simulink model "main_WU_motion"  (R2023a)
settings: Solver=VariableStepAuto  StartTime=0.0  StopTime=3.88  RelTol=1e-9  AbsTol=1e-9  EnableMultiTasking=on
values from neighbouring files (symbols this model uses):
  a_el = [r_ej,h_ej,r_ej]    [data.m]    (also in fo_python_to_matlab.m = [ax,ay,az])
  akt_GH = rand(1,13)*1    [inverse_dynamics.m]    (also in odvozeni_svaly.m = sym('akt_GH',[1 N_GH]))
  akt_ST = rand(1,13)*1    [inverse_dynamics.m]    (also in odvozeni_svaly.m = sym('akt_ST',[1 N_ST]))
  ccom = [-0.0110972, 0.00637508, 0.0541825]    [data.m]    (also in fo_python_to_matlab.m = [ccomx, ccomy, ccomz]; mm_python_to_matlab.m = [ccomx, ccomy, ccomz])
  cI = [5.75482e-05, 6.05521e-05, 1.05345e-05,-1.27405e-05, 1.65861e-05, 4.50136e-06]    [data.m]    (also in mm_python_to_matlab.m = [cixx, ciyy, cizz, cixy, ciyz, cizx])
  cont1 = [-0.083529 -0.01368 -0.098954]-scom    [data.m]    (also in fo_python_to_matlab.m = [x_cont1,y_cont1,z_cont1])
  cont2 = [-0.105456 -0.125076 -0.075251]-scom    [data.m]    (also in fo_python_to_matlab.m = [x_cont2,y_cont2,z_cont2])
  cont_params = [k_contact, eps]    [data.m]    (also in fo_python_to_matlab.m)
  Glenohumeral_F0M = str2double(table2array(GH(:,2)))'    [data.m]
  Glenohumeral_l0 = str2double(table2array(GH(:,3)))'    [data.m]
  h_ej = 0.15    [data.m]
  hcom = [0.000389382, -0.116338, -0.00231072]    [data.m]    (also in fo_python_to_matlab.m = [hcomx, hcomy, hcomz]; mm_python_to_matlab.m = [hcomx, hcomy, hcomz])
  hI = [0.00326632, 4.34807e-05, 0.00325004,-0.000136456, -1.30958e-06, -1.14964e-05]    [data.m]    (also in mm_python_to_matlab.m = [hixx, hiyy, hizz, hixy, hiyz, hizx])
  initialConditions = zeros(1,18)    [inverse_dynamics.m]
  k_contact = 0    [data.m]
  m = [0.0370005,0.12759,0.26363]    [data.m]    (also in fo_python_to_matlab.m = [c_m,s_m,h_m]; mm_python_to_matlab.m = [c_m,s_m,h_m])
  m_el = [x_ej,y_ej,z_ej]    [data.m]    (also in fo_python_to_matlab.m = [mx, my, mz])
  p = [c,k,g]    [data.m]    (also in fo_python_to_matlab.m)
  r_ej = 0.088    [data.m]
  Scapulothoracic_F0M = str2double(table2array(ST(:,2)))'    [data.m]
  Scapulothoracic_l0 = str2double(table2array(ST(:,3)))'    [data.m]
  scom = [-0.0512948, -0.0367122, -0.0430756]    [data.m]    (also in fo_python_to_matlab.m = [scomx, scomy, scomz]; mm_python_to_matlab.m = [scomx, scomy, scomz])
  sI = [0.00020065, 0.000202939, 0.000227237,-4.55661e-05, -7.53511e-05, -7.42694e-05]    [data.m]    (also in mm_python_to_matlab.m = [sixx, siyy, sizz, sixy, siyz, sizx])
  T_c = [-0.01433 0.02007 0.135535]    [data.m]    (also in fo_python_to_matlab.m = [T_cx,T_cy,T_cz]; mm_python_to_matlab.m = [T_cx,T_cy,T_cz]; odvozeni_svaly.m)
  T_d = 1e-20    [data.m]
  T_s = [-0.00955 -0.034 0.009]    [data.m]    (also in fo_python_to_matlab.m = [T_sx,T_sy,T_sz]; mm_python_to_matlab.m = [T_sx,T_sy,T_sz]; odvozeni_svaly.m)
  T_t = [0.006325 0.00693 0.025465]    [data.m]    (also in fo_python_to_matlab.m = [T_tx, T_ty, T_tz]; odvozeni_svaly.m)
  x_ej = -0.03    [data.m]
  y_ej = -0.1    [data.m]
  z_ej = 0.05    [data.m]
undefined symbols (not defined in the file or in its folder): phi_0, r_0, r_10, r_20, X, Y, Z
libraries: sm_lib x165, nesl_utility x96
(part 1 of 5)
settings Model: Creator=zoufi  LastModifiedBy=zoufaond
settings SolverCC: AutoScaleAbsTol=off  AlgebraicLoopSolver=TrustRegion  MaxZcPerStep=1
settings DataIOCC: LimitDataPoints=on  MaxDataPoints=10000
settings OptimizationCC: ReuseModelBlockBuffer=off  LifeSpan=inf
settings DebuggingCC: UnconnectedInputMsg=warning  UnconnectedOutputMsg=warning  UnconnectedLineMsg=warning  AllowSymbolicDim=off  SubsystemReferenceDiagnosticForUnitTest=warning  SFUnexpectedBacktrackingDiag=warning  SFNoUnconditionalDefaultTransitionDiag=warning  SFExecutionAtInitializationDiag=none  ArithmeticOperatorsInVariantConditions=warning
settings ModelReferenceCC: EnableRefExpFcnMdlSchedulingChecks=on
settings SFSimCC: SimUseLocalCustomCode=off  CustomCodeUndefinedFunction=UseInterfaceOnly
settings RTWCC: RTWUseLocalCustomCode=off  DLArmComputeVersion=19.05
settings CodeAppCC: StateflowObjectComments=on
settings GRTTargetCC: TargetLangStandard=C89/C90 (ANSI)
settings ConfigComp: CovMetricSettings=dw  CovSaveCumulativeToWorkspaceVar=on  CovSaveSingleToWorkspaceVar=on  CovExternalEMLEnable=off  CovSFcnEnable=off
settings SimscapeCC: SimscapeLogType=all  SimscapeLogSimulationStatistics=on  SimscapeLogDataHistory=10000

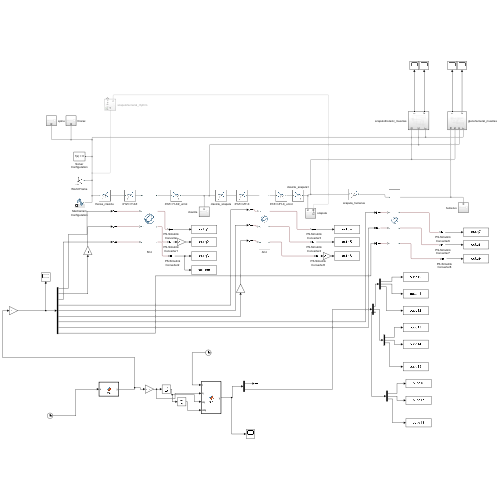
[thumbnail: Simulink's stored preview of the top-level diagram]
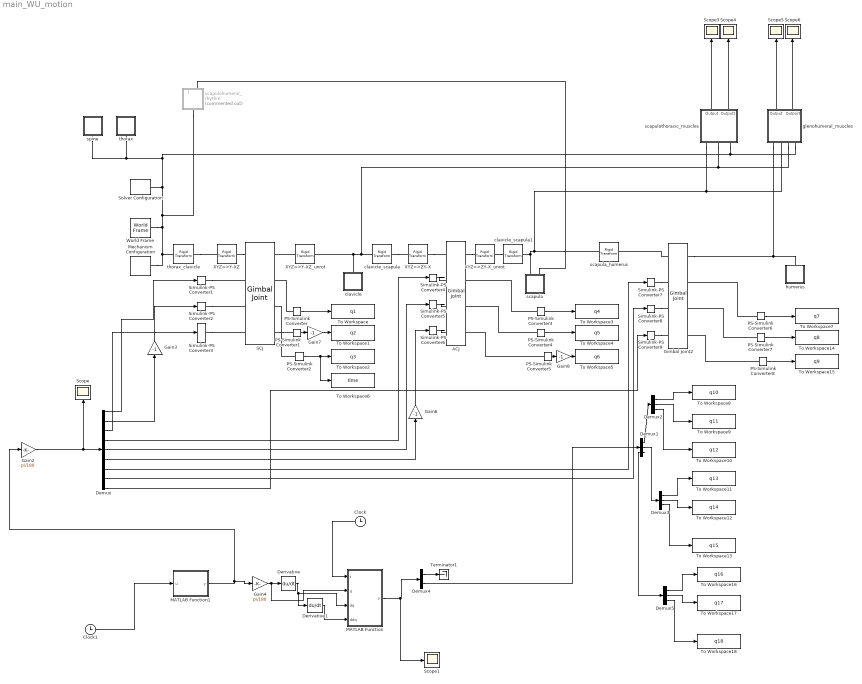
== system main_WU_motion ==
  ACJ : sm_lib/Joints/Gimbal Joint  JointMode=Normal  SenseConstraintForce=off  SenseConstraintForceX=off  SenseConstraintForceY=off  SenseConstraintForceZ=off  SenseConstraintTorque=off  SenseConstraintTorqueX=off  SenseConstraintTorqueY=off  SenseConstraintTorqueZ=off  SenseTotalForce=off  SenseTotalForceX=off  SenseTotalForceY=off  SenseTotalForceZ=off  SenseTotalTorque=off  SenseTotalTorqueX=off  SenseTotalTorqueY=off  SenseTotalTorqueZ=off  CompositeWrenchDir=FollowerOnBase  CompositeWrenchFrame=BaseFrame  RxEquilibriumPosition=0  RxEquilibriumPositionUnits=deg  RxSpringStiffness=k  RxSpringStiffnessUnits=N*m/rad  RxDampingCoefficient=c  RxDampingCoefficientUnits=N*m/(rad/s)  RxTorqueActuationMode=ComputedTorque  RxMotionActuationMode=InputMotion  RxSensePosition=off  RxSenseVelocity=off  RxSenseAcceleration=off  RxSenseTorqueForce=on  RxSenseLowerLimitTorqueForce=off  RxSenseUpperLimitTorqueForce=off  RxLowerLimitSpecify=off  RxLowerLimitBound=-90  RxLowerLimitBoundUnits=deg  RxLowerLimitStiffness=1e4  RxLowerLimitStiffnessUnits=N*m/deg  RxLowerLimitDamping=10  RxLowerLimitDampingUnits=N*m/(deg/s)  RxLowerLimitTransitionRegionWidth=0.1  RxLowerLimitTransitionRegionWidthUnits=deg  RxUpperLimitSpecify=off  RxUpperLimitBound=90  RxUpperLimitBoundUnits=deg  RxUpperLimitStiffness=1e4  RxUpperLimitStiffnessUnits=N*m/deg  RxUpperLimitDamping=10  RxUpperLimitDampingUnits=N*m/(deg/s)  RxUpperLimitTransitionRegionWidth=0.1  RxUpperLimitTransitionRegionWidthUnits=deg  RxPositionTargetSpecify=on  RxPositionTargetPriority=High  RxPositionTargetValue=initialConditions(4)  RxPositionTargetValueUnits=rad  RxVelocityTargetSpecify=off  RxVelocityTargetPriority=High  RxVelocityTargetValue=0  RxVelocityTargetValueUnits=deg/s  RyEquilibriumPosition=0  RyEquilibriumPositionUnits=deg  RySpringStiffness=k  RySpringStiffnessUnits=N*m/rad  RyDampingCoefficient=c  RyDampingCoefficientUnits=N*m/(rad/s)  RyTorqueActuationMode=ComputedTorque  RyMotionActuationMode=InputMotion  RySensePosition=off  RySenseVelocity=off  RySenseAcceleration=off  RySenseTorqueForce=on  RySenseLowerLimitTorqueForce=off  RySenseUpperLimitTorqueForce=off  RyLowerLimitSpecify=off  RyLowerLimitBound=-90  RyLowerLimitBoundUnits=deg  RyLowerLimitStiffness=1e4  RyLowerLimitStiffnessUnits=N*m/deg  RyLowerLimitDamping=10  RyLowerLimitDampingUnits=N*m/(deg/s)  RyLowerLimitTransitionRegionWidth=0.1  RyLowerLimitTransitionRegionWidthUnits=deg  RyUpperLimitSpecify=off  RyUpperLimitBound=90  RyUpperLimitBoundUnits=deg  RyUpperLimitStiffness=1e4  RyUpperLimitStiffnessUnits=N*m/deg  RyUpperLimitDamping=10  RyUpperLimitDampingUnits=N*m/(deg/s)  RyUpperLimitTransitionRegionWidth=0.1  RyUpperLimitTransitionRegionWidthUnits=deg  RyPositionTargetSpecify=on  RyPositionTargetPriority=High  RyPositionTargetValue=initialConditions(5)  RyPositionTargetValueUnits=rad  RyVelocityTargetSpecify=off  RyVelocityTargetPriority=High  RyVelocityTargetValue=0  RyVelocityTargetValueUnits=deg/s  RzEquilibriumPosition=0  RzEquilibriumPositionUnits=deg  RzSpringStiffness=k  RzSpringStiffnessUnits=N*m/rad  RzDampingCoefficient=c  RzDampingCoefficientUnits=N*m/(rad/s)  RzTorqueActuationMode=ComputedTorque  RzMotionActuationMode=InputMotion  RzSensePosition=off  RzSenseVelocity=off  RzSenseAcceleration=off  RzSenseTorqueForce=on  RzSenseLowerLimitTorqueForce=off  RzSenseUpperLimitTorqueForce=off  RzLowerLimitSpecify=off  RzLowerLimitBound=-90  RzLowerLimitBoundUnits=deg  RzLowerLimitStiffness=1e4  RzLowerLimitStiffnessUnits=N*m/deg  RzLowerLimitDamping=10  RzLowerLimitDampingUnits=N*m/(deg/s)  RzLowerLimitTransitionRegionWidth=0.1  RzLowerLimitTransitionRegionWidthUnits=deg  RzUpperLimitSpecify=off  RzUpperLimitBound=90  RzUpperLimitBoundUnits=deg  RzUpperLimitStiffness=1e4  RzUpperLimitStiffnessUnits=N*m/deg  RzUpperLimitDamping=10  RzUpperLimitDampingUnits=N*m/(deg/s)  RzUpperLimitTransitionRegionWidth=0.1  RzUpperLimitTransitionRegionWidthUnits=deg  RzPositionTargetSpecify=on  RzPositionTargetPriority=High  RzPositionTargetValue=initialConditions(6)  RzPositionTargetValueUnits=rad  RzVelocityTargetSpecify=off  RzVelocityTargetPriority=High  RzVelocityTargetValue=0  RzVelocityTargetValueUnits=deg/s
  Clock : Clock
  Clock1 : Clock
  Demux : Demux  Outputs=9
  Demux{1..3,5} (4 alike) : Demux  Outputs=3
  Demux4 : Demux  Outputs=2
  Derivative : Derivative
  Derivative1 : Derivative
  Gain2 : Gain  Gain=pi/180
  Gain{3,6..8} (4 alike) : Gain  Gain=-1
  Gain4 : Gain  Gain=pi/180
  Gimbal Joint2 : sm_lib/Joints/Gimbal Joint  JointMode=Normal  SenseConstraintForce=off  SenseConstraintForceX=off  SenseConstraintForceY=off  SenseConstraintForceZ=off  SenseConstraintTorque=off  SenseConstraintTorqueX=off  SenseConstraintTorqueY=off  SenseConstraintTorqueZ=off  SenseTotalForce=off  SenseTotalForceX=off  SenseTotalForceY=off  SenseTotalForceZ=off  SenseTotalTorque=off  SenseTotalTorqueX=off  SenseTotalTorqueY=off  SenseTotalTorqueZ=off  CompositeWrenchDir=FollowerOnBase  CompositeWrenchFrame=BaseFrame  RxEquilibriumPosition=0  RxEquilibriumPositionUnits=deg  RxSpringStiffness=k  RxSpringStiffnessUnits=N*m/rad  RxDampingCoefficient=c  RxDampingCoefficientUnits=N*m/(rad/s)  RxTorqueActuationMode=ComputedTorque  RxMotionActuationMode=InputMotion  RxSensePosition=off  RxSenseVelocity=off  RxSenseAcceleration=off  RxSenseTorqueForce=on  RxSenseLowerLimitTorqueForce=off  RxSenseUpperLimitTorqueForce=off  RxLowerLimitSpecify=off  RxLowerLimitBound=-90  RxLowerLimitBoundUnits=deg  RxLowerLimitStiffness=1e4  RxLowerLimitStiffnessUnits=N*m/deg  RxLowerLimitDamping=10  RxLowerLimitDampingUnits=N*m/(deg/s)  RxLowerLimitTransitionRegionWidth=0.1  RxLowerLimitTransitionRegionWidthUnits=deg  RxUpperLimitSpecify=off  RxUpperLimitBound=90  RxUpperLimitBoundUnits=deg  RxUpperLimitStiffness=1e4  RxUpperLimitStiffnessUnits=N*m/deg  RxUpperLimitDamping=10  RxUpperLimitDampingUnits=N*m/(deg/s)  RxUpperLimitTransitionRegionWidth=0.1  RxUpperLimitTransitionRegionWidthUnits=deg  RxPositionTargetSpecify=on  RxPositionTargetPriority=High  RxPositionTargetValue=initialConditions(4)  RxPositionTargetValueUnits=rad  RxVelocityTargetSpecify=off  RxVelocityTargetPriority=High  RxVelocityTargetValue=0  RxVelocityTargetValueUnits=deg/s  RyEquilibriumPosition=0  RyEquilibriumPositionUnits=deg  RySpringStiffness=k  RySpringStiffnessUnits=N*m/rad  RyDampingCoefficient=c  RyDampingCoefficientUnits=N*m/(rad/s)  RyTorqueActuationMode=ComputedTorque  RyMotionActuationMode=InputMotion  RySensePosition=off  RySenseVelocity=off  RySenseAcceleration=off  RySenseTorqueForce=on  RySenseLowerLimitTorqueForce=off  RySenseUpperLimitTorqueForce=off  RyLowerLimitSpecify=off  RyLowerLimitBound=-90  RyLowerLimitBoundUnits=deg  RyLowerLimitStiffness=1e4  RyLowerLimitStiffnessUnits=N*m/deg  RyLowerLimitDamping=10  RyLowerLimitDampingUnits=N*m/(deg/s)  RyLowerLimitTransitionRegionWidth=0.1  RyLowerLimitTransitionRegionWidthUnits=deg  RyUpperLimitSpecify=off  RyUpperLimitBound=90  RyUpperLimitBoundUnits=deg  RyUpperLimitStiffness=1e4  RyUpperLimitStiffnessUnits=N*m/deg  RyUpperLimitDamping=10  RyUpperLimitDampingUnits=N*m/(deg/s)  RyUpperLimitTransitionRegionWidth=0.1  RyUpperLimitTransitionRegionWidthUnits=deg  RyPositionTargetSpecify=on  RyPositionTargetPriority=High  RyPositionTargetValue=initialConditions(5)  RyPositionTargetValueUnits=rad  RyVelocityTargetSpecify=off  RyVelocityTargetPriority=High  RyVelocityTargetValue=0  RyVelocityTargetValueUnits=deg/s  RzEquilibriumPosition=0  RzEquilibriumPositionUnits=deg  RzSpringStiffness=k  RzSpringStiffnessUnits=N*m/rad  RzDampingCoefficient=c  RzDampingCoefficientUnits=N*m/(rad/s)  RzTorqueActuationMode=ComputedTorque  RzMotionActuationMode=InputMotion  RzSensePosition=off  RzSenseVelocity=off  RzSenseAcceleration=off  RzSenseTorqueForce=on  RzSenseLowerLimitTorqueForce=off  RzSenseUpperLimitTorqueForce=off  RzLowerLimitSpecify=off  RzLowerLimitBound=-90  RzLowerLimitBoundUnits=deg  RzLowerLimitStiffness=1e4  RzLowerLimitStiffnessUnits=N*m/deg  RzLowerLimitDamping=10  RzLowerLimitDampingUnits=N*m/(deg/s)  RzLowerLimitTransitionRegionWidth=0.1  RzLowerLimitTransitionRegionWidthUnits=deg  RzUpperLimitSpecify=off  RzUpperLimitBound=90  RzUpperLimitBoundUnits=deg  RzUpperLimitStiffness=1e4  RzUpperLimitStiffnessUnits=N*m/deg  RzUpperLimitDamping=10  RzUpperLimitDampingUnits=N*m/(deg/s)  RzUpperLimitTransitionRegionWidth=0.1  RzUpperLimitTransitionRegionWidthUnits=deg  RzPositionTargetSpecify=on  RzPositionTargetPriority=High  RzPositionTargetValue=initialConditions(6)  RzPositionTargetValueUnits=rad  RzVelocityTargetSpecify=off  RzVelocityTargetPriority=High  RzVelocityTargetValue=0  RzVelocityTargetValueUnits=deg/s
  MATLAB Function : MATLAB Function  TreatAsAtomicUnit=on
  MATLAB Function1 : MATLAB Function  TreatAsAtomicUnit=on
  Mechanism Configuration : sm_lib/Utilities/Mechanism Configuration  UniformGravity=Constant  GravityVector=[0 -9.80665 0]  GravityVectorUnits=m/s^2  LinearizationDelta=0.001  JointModeTransitionNonlinearIterations=2
  PS-Simulink Converter{,1..8} (9 alike) : nesl_utility/PS-Simulink Converter  PhysicalDomain=network_engine_domain  SubClassName=ps_output  LeftPortType=input  RightPortType=output  PseudoPeriodic=off  Frequencies=[]  VectorFormat=inherit  Unit=inherit  AffineConversion=off
  SCJ : sm_lib/Joints/Gimbal Joint  JointMode=Normal  SenseConstraintForce=off  SenseConstraintForceX=off  SenseConstraintForceY=off  SenseConstraintForceZ=off  SenseConstraintTorque=off  SenseConstraintTorqueX=off  SenseConstraintTorqueY=off  SenseConstraintTorqueZ=off  SenseTotalForce=off  SenseTotalForceX=off  SenseTotalForceY=off  SenseTotalForceZ=off  SenseTotalTorque=off  SenseTotalTorqueX=off  SenseTotalTorqueY=off  SenseTotalTorqueZ=off  CompositeWrenchDir=FollowerOnBase  CompositeWrenchFrame=BaseFrame  RxEquilibriumPosition=0  RxEquilibriumPositionUnits=deg  RxSpringStiffness=k  RxSpringStiffnessUnits=N*m/rad  RxDampingCoefficient=c  RxDampingCoefficientUnits=N*m/(rad/s)  RxTorqueActuationMode=ComputedTorque  RxMotionActuationMode=InputMotion  RxSensePosition=off  RxSenseVelocity=off  RxSenseAcceleration=off  RxSenseTorqueForce=on  RxSenseLowerLimitTorqueForce=off  RxSenseUpperLimitTorqueForce=off  RxLowerLimitSpecify=off  RxLowerLimitBound=-90  RxLowerLimitBoundUnits=deg  RxLowerLimitStiffness=1e4  RxLowerLimitStiffnessUnits=N*m/deg  RxLowerLimitDamping=10  RxLowerLimitDampingUnits=N*m/(deg/s)  RxLowerLimitTransitionRegionWidth=0.1  RxLowerLimitTransitionRegionWidthUnits=deg  RxUpperLimitSpecify=off  RxUpperLimitBound=90  RxUpperLimitBoundUnits=deg  RxUpperLimitStiffness=1e4  RxUpperLimitStiffnessUnits=N*m/deg  RxUpperLimitDamping=10  RxUpperLimitDampingUnits=N*m/(deg/s)  RxUpperLimitTransitionRegionWidth=0.1  RxUpperLimitTransitionRegionWidthUnits=deg  RxPositionTargetSpecify=on  RxPositionTargetPriority=High  RxPositionTargetValue=initialConditions(1)  RxPositionTargetValueUnits=rad  RxVelocityTargetSpecify=off  RxVelocityTargetPriority=High  RxVelocityTargetValue=0  RxVelocityTargetValueUnits=deg/s  RyEquilibriumPosition=0  RyEquilibriumPositionUnits=deg  RySpringStiffness=k  RySpringStiffnessUnits=N*m/rad  RyDampingCoefficient=c  RyDampingCoefficientUnits=N*m/(rad/s)  RyTorqueActuationMode=ComputedTorque  RyMotionActuationMode=InputMotion  RySensePosition=off  RySenseVelocity=off  RySenseAcceleration=off  RySenseTorqueForce=on  RySenseLowerLimitTorqueForce=off  RySenseUpperLimitTorqueForce=off  RyLowerLimitSpecify=off  RyLowerLimitBound=-90  RyLowerLimitBoundUnits=deg  RyLowerLimitStiffness=1e4  RyLowerLimitStiffnessUnits=N*m/deg  RyLowerLimitDamping=10  RyLowerLimitDampingUnits=N*m/(deg/s)  RyLowerLimitTransitionRegionWidth=0.1  RyLowerLimitTransitionRegionWidthUnits=deg  RyUpperLimitSpecify=off  RyUpperLimitBound=90  RyUpperLimitBoundUnits=deg  RyUpperLimitStiffness=1e4  RyUpperLimitStiffnessUnits=N*m/deg  RyUpperLimitDamping=10  RyUpperLimitDampingUnits=N*m/(deg/s)  RyUpperLimitTransitionRegionWidth=0.1  RyUpperLimitTransitionRegionWidthUnits=deg  RyPositionTargetSpecify=on  RyPositionTargetPriority=High  RyPositionTargetValue=initialConditions(2)  RyPositionTargetValueUnits=rad  RyVelocityTargetSpecify=off  RyVelocityTargetPriority=High  RyVelocityTargetValue=0  RyVelocityTargetValueUnits=deg/s  RzEquilibriumPosition=0  RzEquilibriumPositionUnits=deg  RzSpringStiffness=k  RzSpringStiffnessUnits=N*m/rad  RzDampingCoefficient=c  RzDampingCoefficientUnits=N*m/(rad/s)  RzTorqueActuationMode=ComputedTorque  RzMotionActuationMode=InputMotion  RzSensePosition=off  RzSenseVelocity=off  RzSenseAcceleration=off  RzSenseTorqueForce=on  RzSenseLowerLimitTorqueForce=off  RzSenseUpperLimitTorqueForce=off  RzLowerLimitSpecify=off  RzLowerLimitBound=-90  RzLowerLimitBoundUnits=deg  RzLowerLimitStiffness=1e4  RzLowerLimitStiffnessUnits=N*m/deg  RzLowerLimitDamping=10  RzLowerLimitDampingUnits=N*m/(deg/s)  RzLowerLimitTransitionRegionWidth=0.1  RzLowerLimitTransitionRegionWidthUnits=deg  RzUpperLimitSpecify=off  RzUpperLimitBound=90  RzUpperLimitBoundUnits=deg  RzUpperLimitStiffness=1e4  RzUpperLimitStiffnessUnits=N*m/deg  RzUpperLimitDamping=10  RzUpperLimitDampingUnits=N*m/(deg/s)  RzUpperLimitTransitionRegionWidth=0.1  RzUpperLimitTransitionRegionWidthUnits=deg  RzPositionTargetSpecify=on  RzPositionTargetPriority=High  RzPositionTargetValue=initialConditions(3)  RzPositionTargetValueUnits=rad  RzVelocityTargetSpecify=off  RzVelocityTargetPriority=High  RzVelocityTargetValue=0  RzVelocityTargetValueUnits=deg/s
  Scope{,1,3..6} (6 alike) : Scope
  Simulink-PS Converter{1..2,4..9} (8 alike) : nesl_utility/Simulink-PS Converter  PhysicalDomain=network_engine_domain  SubClassName=ps_input  LeftPortType=input  RightPortType=output  PseudoPeriodic=off  Frequencies=[]  NoiseDistribution=none  NoiseParameters=[]  Unit=1  AffineConversion=off  FilteringAndDerivatives=filter  SimscapeFilterOrder=2  InputFilterTimeConstant=0.001  UdotUserProvided=0
  Simulink-PS Converter3 : nesl_utility/Simulink-PS Converter  PhysicalDomain=network_engine_domain  SubClassName=ps_input  LeftPortType=input  RightPortType=output  PseudoPeriodic=off  Frequencies=[]  NoiseDistribution=none  NoiseParameters=[]  Unit=1  AffineConversion=off  FilteringAndDerivatives=filter  SimscapeFilterOrder=2  InputFilterTimeConstant=0.001  UdotUserProvided=2
  Solver Configuration : nesl_utility/Solver Configuration  PhysicalDomain=network_engine_domain  SubClassName=solver  LeftPortType=input  RightPortType=generic  Tones=[]  Harmonics=[]  SimulateNoise=off  Profile=off  UseLocalSampling=off  EnableSwitchedLinearOptims=on  FrequencyDomain=off  UseCCode=off  RelTol=0.001  AbsTol=1e-06  MinStep=1e-09  ToWorkspace=off  RevertToSquareIcSolve=off  NumHomotopyIterations=100  PhasorMode=off  PhasorModeNumHarmonics=1  ConsistencySolver=NEWTON_XTOL_AFTER_FTOL  IndexReductionMethod=DerivativeReplacement  DoDC=off  ResidualTolerance=1e-09  ConsistencyTolSource=GLOBAL  ConsistencyAbsTol=0.001  ConsistencyRelTol=0.001  ConsistencyTolFactor=0.001  UseLocalSolver=off  LocalSolverChoice=NE_BACKWARD_EULER_ADVANCER  ResolveIndetEquations=on  FunctionEvalNumThread=1  LocalSolverSampleTime=0.001  DoFixedCost=off  MaxNonlinIter=3  MaxModeIter=2  ComputeImpulses=off  ImpulseIterations=2  LinearAlgebra=Sparse  LinearAlgebraNumThread=0  EquationFormulation=NE_TIME_EF  DelaysMemoryBudget=1024  AutomaticFiltering=on  FilteringTimeConstant=0.001  PartitionStorageMethod=AS_NEEDED  PartitionMemoryBudget=1024  PartitionMethod=FAST
  Terminator1 : Terminator
  To Workspace : ToWorkspace  VariableName=q1  SampleTime=-1
  To Workspace1 : ToWorkspace  VariableName=q2  SampleTime=-1
  To Workspace10 : ToWorkspace  VariableName=q12  SampleTime=-1
  To Workspace11 : ToWorkspace  VariableName=q13  SampleTime=-1
  To Workspace12 : ToWorkspace  VariableName=q14  SampleTime=-1
  To Workspace13 : ToWorkspace  VariableName=q15  SampleTime=-1
  To Workspace14 : ToWorkspace  VariableName=q8  SampleTime=-1
  To Workspace15 : ToWorkspace  VariableName=q9  SampleTime=-1
  To Workspace16 : ToWorkspace  VariableName=q16  SampleTime=-1
  To Workspace17 : ToWorkspace  VariableName=q17  SampleTime=-1
  To Workspace18 : ToWorkspace  VariableName=q18  SampleTime=-1
  To Workspace2 : ToWorkspace  VariableName=q3  SampleTime=-1
  To Workspace3 : ToWorkspace  VariableName=q4  SampleTime=-1
  To Workspace4 : ToWorkspace  VariableName=q5  SampleTime=-1
  To Workspace5 : ToWorkspace  VariableName=q6  SampleTime=-1
  To Workspace6 : ToWorkspace  VariableName=time  SaveFormat=Structure With Time  SampleTime=-1
  To Workspace7 : ToWorkspace  VariableName=q7  SampleTime=-1
  To Workspace8 : ToWorkspace  VariableName=q10  SampleTime=-1
  To Workspace9 : ToWorkspace  VariableName=q11  SampleTime=-1
  World Frame : sm_lib/Frames and Transforms/World Frame
  XYZ=>Y-XZ : sm_lib/Frames and Transforms/Rigid Transform  TranslationMethod=None  TranslationStandardOffset=0  TranslationStandardOffsetUnits=m  TranslationStandardAxis=+Z  TranslationCartesianOffset=T_t  TranslationCartesianOffsetUnits=m  TranslationROffset=0  TranslationROffsetUnits=m  TranslationZOffset=0  TranslationZOffsetUnits=m  TranslationThetaOffset=0  TranslationThetaOffsetUnits=deg  RotationMethod=StandardAxis  RotationAngleUnits=deg  RotationStandardAxis=+Z  RotationAngle=90  RotationArbitraryAxis=[0 0 1]  FollAlignAxisA=+X  BaseAlignAxisA=+Y  FollAlignAxisB=+Y  BaseAlignAxisB=+Z  RotationSequenceAxes=FollowerAxes  RotationSequence=XYX  RotationSequenceAngles=[0 0 0]  RotationSequenceAnglesUnits=deg  RotationMatrix=[1 0 0; 0 1 0; 0 0 1]  Quaternion=[1 0 0 0]
  XYZ=>Y-XZ_unrot : sm_lib/Frames and Transforms/Rigid Transform  TranslationMethod=None  TranslationStandardOffset=0  TranslationStandardOffsetUnits=m  TranslationStandardAxis=+Z  TranslationCartesianOffset=T_t  TranslationCartesianOffsetUnits=m  TranslationROffset=0  TranslationROffsetUnits=m  TranslationZOffset=0  TranslationZOffsetUnits=m  TranslationThetaOffset=0  TranslationThetaOffsetUnits=deg  RotationMethod=StandardAxis  RotationAngleUnits=deg  RotationStandardAxis=+Z  RotationAngle=90  RotationArbitraryAxis=[0 0 1]  FollAlignAxisA=+X  BaseAlignAxisA=+Y  FollAlignAxisB=+Y  BaseAlignAxisB=+Z  RotationSequenceAxes=FollowerAxes  RotationSequence=XYX  RotationSequenceAngles=[0 0 0]  RotationSequenceAnglesUnits=deg  RotationMatrix=[1 0 0; 0 1 0; 0 0 1]  Quaternion=[1 0 0 0]
  XYZ=>ZY-X : sm_lib/Frames and Transforms/Rigid Transform  TranslationMethod=None  TranslationStandardOffset=0  TranslationStandardOffsetUnits=m  TranslationStandardAxis=+Z  TranslationCartesianOffset=[0 0 0]  TranslationCartesianOffsetUnits=m  TranslationROffset=0  TranslationROffsetUnits=m  TranslationZOffset=0  TranslationZOffsetUnits=m  TranslationThetaOffset=0  TranslationThetaOffsetUnits=deg  RotationMethod=StandardAxis  RotationAngleUnits=deg  RotationStandardAxis=-Y  RotationAngle=90  RotationArbitraryAxis=[0 0 1]  FollAlignAxisA=+X  BaseAlignAxisA=+Y  FollAlignAxisB=+Y  BaseAlignAxisB=+Z  RotationSequenceAxes=FollowerAxes  RotationSequence=XYX  RotationSequenceAngles=[90 -90 0]  RotationSequenceAnglesUnits=deg  RotationMatrix=[1 0 0; 0 1 0; 0 0 1]  Quaternion=[1 0 0 0]
  XYZ=>ZY-X_unrot : sm_lib/Frames and Transforms/Rigid Transform  TranslationMethod=None  TranslationStandardOffset=0  TranslationStandardOffsetUnits=m  TranslationStandardAxis=+Z  TranslationCartesianOffset=[0 0 0]  TranslationCartesianOffsetUnits=m  TranslationROffset=0  TranslationROffsetUnits=m  TranslationZOffset=0  TranslationZOffsetUnits=m  TranslationThetaOffset=0  TranslationThetaOffsetUnits=deg  RotationMethod=StandardAxis  RotationAngleUnits=deg  RotationStandardAxis=-Y  RotationAngle=90  RotationArbitraryAxis=[0 0 1]  FollAlignAxisA=+X  BaseAlignAxisA=+Y  FollAlignAxisB=+Y  BaseAlignAxisB=+Z  RotationSequenceAxes=FollowerAxes  RotationSequence=XYX  RotationSequenceAngles=[90 -90 0]  RotationSequenceAnglesUnits=deg  RotationMatrix=[1 0 0; 0 1 0; 0 0 1]  Quaternion=[1 0 0 0]
  clavicle : Subsystem
  clavicle_scapula : sm_lib/Frames and Transforms/Rigid Transform  TranslationMethod=Cartesian  TranslationStandardOffset=0  TranslationStandardOffsetUnits=m  TranslationStandardAxis=+Z  TranslationCartesianOffset=T_c  TranslationCartesianOffsetUnits=m  TranslationROffset=0  TranslationROffsetUnits=m  TranslationZOffset=0  TranslationZOffsetUnits=m  TranslationThetaOffset=0  TranslationThetaOffsetUnits=deg  RotationMethod=RotationSequence  RotationAngleUnits=deg  RotationStandardAxis=+Z  RotationAngle=0.0  RotationArbitraryAxis=[0 0 1]  FollAlignAxisA=+X  BaseAlignAxisA=+Y  FollAlignAxisB=+Y  BaseAlignAxisB=+Z  RotationSequenceAxes=FollowerAxes  RotationSequence=XYZ  RotationSequenceAngles=[-0.52 0.52 0]  RotationSequenceAnglesUnits=rad  RotationMatrix=[1 0 0; 0 1 0; 0 0 1]  Quaternion=[1 0 0 0]
  clavicle_scapula1 : sm_lib/Frames and Transforms/Rigid Transform  TranslationMethod=None  TranslationStandardOffset=0  TranslationStandardOffsetUnits=m  TranslationStandardAxis=+Z  TranslationCartesianOffset=T_c  TranslationCartesianOffsetUnits=m  TranslationROffset=0  TranslationROffsetUnits=m  TranslationZOffset=0  TranslationZOffsetUnits=m  TranslationThetaOffset=0  TranslationThetaOffsetUnits=deg  RotationMethod=RotationSequence  RotationAngleUnits=deg  RotationStandardAxis=+Z  RotationAngle=0.0  RotationArbitraryAxis=[0 0 1]  FollAlignAxisA=+X  BaseAlignAxisA=+Y  FollAlignAxisB=+Y  BaseAlignAxisB=+Z  RotationSequenceAxes=FollowerAxes  RotationSequence=XYZ  RotationSequenceAngles=[-0.52 0.52 0]  RotationSequenceAnglesUnits=rad  RotationMatrix=[1 0 0; 0 1 0; 0 0 1]  Quaternion=[1 0 0 0]
  glenohumeral_muscles : Subsystem
  humerus : Subsystem
  scapula : Subsystem
  scapula_humerus : sm_lib/Frames and Transforms/Rigid Transform  TranslationMethod=Cartesian  TranslationStandardOffset=0  TranslationStandardOffsetUnits=m  TranslationStandardAxis=+Z  TranslationCartesianOffset=T_s  TranslationCartesianOffsetUnits=m  TranslationROffset=0  TranslationROffsetUnits=m  TranslationZOffset=0  TranslationZOffsetUnits=m  TranslationThetaOffset=0  TranslationThetaOffsetUnits=deg  RotationMethod=None  RotationAngleUnits=deg  RotationStandardAxis=+Z  RotationAngle=0.0  RotationArbitraryAxis=[0 0 1]  FollAlignAxisA=+X  BaseAlignAxisA=+Y  FollAlignAxisB=+Y  BaseAlignAxisB=+Z  RotationSequenceAxes=FollowerAxes  RotationSequence=XYX  RotationSequenceAngles=[0 0 0]  RotationSequenceAnglesUnits=deg  RotationMatrix=[1 0 0; 0 1 0; 0 0 1]  Quaternion=[1 0 0 0]
  scapulohumeral_rhythm : Subsystem  Commented=on
  scapulothoracic_muscles : Subsystem
  spine : Subsystem
  thorax : Subsystem
  thorax_clavicle : sm_lib/Frames and Transforms/Rigid Transform  TranslationMethod=Cartesian  TranslationStandardOffset=0  TranslationStandardOffsetUnits=m  TranslationStandardAxis=+Z  TranslationCartesianOffset=T_t  TranslationCartesianOffsetUnits=m  TranslationROffset=0  TranslationROffsetUnits=m  TranslationZOffset=0  TranslationZOffsetUnits=m  TranslationThetaOffset=0  TranslationThetaOffsetUnits=deg  RotationMethod=None  RotationAngleUnits=deg  RotationStandardAxis=+Z  RotationAngle=90  RotationArbitraryAxis=[0 0 1]  FollAlignAxisA=+X  BaseAlignAxisA=+Y  FollAlignAxisB=+Y  BaseAlignAxisB=+Z  RotationSequenceAxes=FollowerAxes  RotationSequence=XYX  RotationSequenceAngles=[0 0 0]  RotationSequenceAnglesUnits=deg  RotationMatrix=[1 0 0; 0 1 0; 0 0 1]  Quaternion=[1 0 0 0]
  wires:
  PS-Simulink Converter/1 -> To Workspace/1
  PS-Simulink Converter2/1 -> To Workspace6/1, To Workspace2/1
  PS-Simulink Converter4/1 -> To Workspace4/1
  PS-Simulink Converter3/1 -> To Workspace3/1
  Demux1/1 -> Demux2/1
  Demux2/1 -> To Workspace8/1
  Demux2/2 -> To Workspace9/1
  Demux2/3 -> To Workspace10/1
  Demux1/2 -> Demux3/1
  Demux3/1 -> To Workspace11/1
  Demux3/2 -> To Workspace12/1
  Demux3/3 -> To Workspace13/1
  MATLAB Function/1(y) -> Scope1/1, Demux4/1
  Demux4/1 -> Terminator1/1
  Demux4/2 -> Demux1/1
  PS-Simulink Converter6/1 -> To Workspace7/1
  PS-Simulink Converter7/1 -> To Workspace14/1
  PS-Simulink Converter8/1 -> To Workspace15/1
  Demux5/3 -> To Workspace18/1
  Demux5/2 -> To Workspace17/1
  Demux5/1 -> To Workspace16/1
  Demux1/3 -> Demux5/1
  Derivative/1 -> Derivative1/1, MATLAB Function/3(dq)
  Derivative1/1 -> MATLAB Function/4(ddq)
  glenohumeral_muscles/1(Output) -> Scope5/1
  glenohumeral_muscles/2(Outport) -> Scope6/1
  scapulothoracic_muscles/1(Output) -> Scope3/1
  scapulothoracic_muscles/2(Output1) -> Scope4/1
  MATLAB Function1/1(y) -> Gain2/1, Gain4/1
  Demux/3 -> Simulink-PS Converter3/1
  Demux/7 -> Simulink-PS Converter7/1
  Demux/9 -> Simulink-PS Converter9/1
  Gain2/1 -> Scope/1, Demux/1
  Demux/2 -> Gain3/1
  Gain3/1 -> Simulink-PS Converter2/1
  Demux/4 -> Simulink-PS Converter4/1
  Demux/5 -> Simulink-PS Converter5/1
  Demux/6 -> Gain6/1
  Demux/1 -> Simulink-PS Converter1/1
  Clock/1 -> MATLAB Function/1(t)
  Clock1/1 -> MATLAB Function1/1(u)
  Gain4/1 -> MATLAB Function/2(q), Derivative/1
  PS-Simulink Converter1/1 -> Gain7/1
  Gain7/1 -> To Workspace1/1
  Gain8/1 -> To Workspace5/1
  PS-Simulink Converter5/1 -> Gain8/1
  Gain6/1 -> Simulink-PS Converter6/1
  Demux/8 -> Simulink-PS Converter8/1
  connections:
  PS-Simulink Converter/LConn1 -- SCJ/RConn2
  PS-Simulink Converter1/LConn1 -- SCJ/RConn3
  PS-Simulink Converter2/LConn1 -- SCJ/RConn4
  PS-Simulink Converter5/LConn1 -- ACJ/RConn4
  PS-Simulink Converter4/LConn1 -- ACJ/RConn3
  PS-Simulink Converter3/LConn1 -- ACJ/RConn2
  World Frame/RConn1 -- scapulohumeral_rhythm/LConn1 -- thorax/LConn1 -- spine/LConn1 -- scapulothoracic_muscles/LConn3 -- glenohumeral_muscles/LConn4 -- Solver Configuration/RConn1 -- Mechanism Configuration/RConn1 -- thorax_clavicle/LConn1
  Gimbal Joint2/RConn1 -- glenohumeral_muscles/LConn1 -- humerus/LConn1
  PS-Simulink Converter6/LConn1 -- Gimbal Joint2/RConn2
  PS-Simulink Converter7/LConn1 -- Gimbal Joint2/RConn3
  PS-Simulink Converter8/LConn1 -- Gimbal Joint2/RConn4
  Gimbal Joint2/LConn1 -- scapula_humerus/RConn1
  XYZ=>Y-XZ/RConn1 -- SCJ/LConn1
  scapula/RConn2 -- scapulohumeral_rhythm/RConn1
  Simulink-PS Converter1/RConn1 -- SCJ/LConn2
  Simulink-PS Converter2/RConn1 -- SCJ/LConn3
  Simulink-PS Converter3/RConn1 -- SCJ/LConn4
  Simulink-PS Converter4/RConn1 -- ACJ/LConn2
  Simulink-PS Converter5/RConn1 -- ACJ/LConn3
  Simulink-PS Converter6/RConn1 -- ACJ/LConn4
  Simulink-PS Converter7/RConn1 -- Gimbal Joint2/LConn2
  Simulink-PS Converter8/RConn1 -- Gimbal Joint2/LConn3
  Simulink-PS Converter9/RConn1 -- Gimbal Joint2/LConn4
  clavicle_scapula1/LConn1 -- scapulothoracic_muscles/LConn1 -- glenohumeral_muscles/LConn2 -- scapula_humerus/LConn1 -- scapula/RConn1
  XYZ=>ZY-X_unrot/LConn1 -- clavicle_scapula1/RConn1
  scapulothoracic_muscles/LConn2 -- glenohumeral_muscles/LConn3 -- clavicle_scapula/LConn1 -- XYZ=>Y-XZ_unrot/LConn1 -- clavicle/LConn1
  clavicle_scapula/RConn1 -- XYZ=>ZY-X/LConn1
  thorax_clavicle/RConn1 -- XYZ=>Y-XZ/LConn1
  XYZ=>Y-XZ_unrot/RConn1 -- SCJ/RConn1
  XYZ=>ZY-X/RConn1 -- ACJ/LConn1
  ACJ/RConn1 -- XYZ=>ZY-X_unrot/RConn1

== system main_WU_motion/clavicle ==
  body : sm_lib/Body Elements/File Solid  ExtGeomFileName=bones/clavicle.obj  UnitType=Custom  ExtGeomFileUnits=m  StepReaderType=HEX  ExportConvexHullGeometry=off  InertiaType=Custom  Mass=m(1)  MassUnits=kg  CenterOfMass=ccom  CenterOfMassUnits=m  MomentsOfInertia=cI(1:3)  MomentsOfInertiaUnits=kg*m^2  ProductsOfInertia=cI(4:6)  ProductsOfInertiaUnits=kg*m^2  BasedOnType=Density  Density=1850  DensityUnits=kg/m^3  DoExposeReferenceFrame=on  SerializedFrames=<Frames/>  GraphicType=FromGeometry  MarkerShape=Sphere  MarkerSize=10  GraphicVisPropType=SimpleVisualProperties  GraphicDiffuseColor=[0.5 0.5 0.5]  GraphicSpecularColor=[0.5 0.5 0.5 1.0]  GraphicAmbientColor=[0.15 0.15 0.15 1.0]  GraphicEmissiveColor=[0.0 0.0 0.0 1.0]  GraphicShininess=75  GraphicOpacity=1.0
  C : PMIOPort  Side=Left
  connections:
  C/RConn1 -- body/RConn1

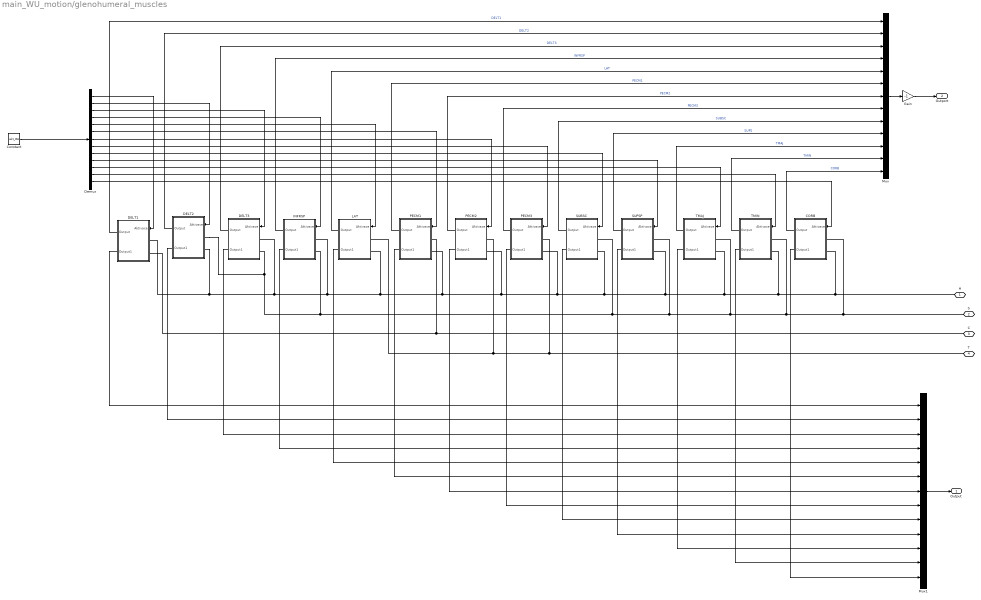
== system main_WU_motion/glenohumeral_muscles ==
  CORB : Subsystem
  Constant : Constant  Value=akt_GH
  DELT1 : Subsystem
  DELT2 : Subsystem
  DELT3 : Subsystem
  Demux : Demux  Outputs=13
  Gain : Gain  Gain=-1
  INFRSP : Subsystem
  LAT : Subsystem
  Mux : Mux  Inputs=13
  Mux1 : Mux  Inputs=13
  PECM1 : Subsystem
  PECM2 : Subsystem
  PECM3 : Subsystem
  SUBSC : Subsystem
  SUPSP : Subsystem
  TMAJ : Subsystem
  TMIN : Subsystem
  H : PMIOPort  Side=Left
  S : PMIOPort  Port=2  Side=Left
  C : PMIOPort  Port=3  Side=Left
  T : PMIOPort  Port=4  Side=Left
  Output : Outport
  Outport : Outport  Port=2
  wires:
  SUPSP/2(Output1) -> Mux1/10
  PECM2/2(Output1) -> Mux1/7
  DELT1/1(Output) -> Mux/1  "DELT1"
  LAT/2(Output1) -> Mux1/5
  DELT2/1(Output) -> Mux/2  "DELT2"
  SUPSP/1(Output) -> Mux/10  "SUPS"
  SUBSC/2(Output1) -> Mux1/9
  CORB/2(Output1) -> Mux1/13
  PECM1/1(Output) -> Mux/6  "PECM1"
  LAT/1(Output) -> Mux/5  "LAT"
  DELT2/2(Output1) -> Mux1/2
  INFRSP/1(Output) -> Mux/4  "INFRSP"
  TMIN/2(Output1) -> Mux1/12
  INFRSP/2(Output1) -> Mux1/4
  TMAJ/1(Output) -> Mux/11  "TMAJ"
  DELT3/2(Output1) -> Mux1/3
  DELT3/1(Output) -> Mux/3  "DELT3"
  PECM2/1(Output) -> Mux/7  "PECM2"
  Mux/1 -> Gain/1
  DELT1/2(Output1) -> Mux1/1
  SUBSC/1(Output) -> Mux/9  "SUBSC"
  TMIN/1(Output) -> Mux/12  "TMIN"
  CORB/1(Output) -> Mux/13  "CORB"
  TMAJ/2(Output1) -> Mux1/11
  PECM1/2(Output1) -> Mux1/6
  PECM3/1(Output) -> Mux/8  "PECM3"
  PECM3/2(Output1) -> Mux1/8
  Mux1/1 -> Output/1
  Gain/1 -> Outport/1
  Demux/1 -> DELT1/1(Aktivace)
  Demux/2 -> DELT2/1(Aktivace)
  Demux/3 -> DELT3/1(Aktivace)
  Demux/4 -> INFRSP/1(Aktivace)
  Demux/5 -> LAT/1(Aktivace)
  Demux/6 -> PECM1/1(Aktivace)
  Demux/7 -> PECM2/1(Aktivace)
  Demux/8 -> PECM3/1(Aktivace)
  Demux/9 -> SUBSC/1(Aktivace)
  Demux/10 -> SUPSP/1(Aktivace)
  Demux/11 -> TMAJ/1(Aktivace)
  Demux/12 -> TMIN/1(Aktivace)
  Demux/13 -> CORB/1(Aktivace)
  Constant/1 -> Demux/1
  connections:
  DELT1/LConn1 -- SUPSP/LConn2 -- H/RConn1 -- CORB/LConn2 -- TMIN/LConn2 -- TMAJ/LConn2 -- SUBSC/LConn2 -- PECM3/LConn2 -- PECM2/LConn2 -- PECM1/LConn2 -- LAT/LConn2 -- INFRSP/LConn1 -- DELT3/LConn1 -- DELT2/LConn2
  DELT1/LConn2 -- C/RConn1 -- PECM1/LConn1
  SUBSC/LConn1 -- S/RConn1 -- CORB/LConn1 -- TMIN/LConn1 -- TMAJ/LConn1 -- SUPSP/LConn1 -- INFRSP/LConn2 -- DELT3/LConn2 -- DELT2/LConn1
  LAT/LConn1 -- T/RConn1 -- PECM3/LConn1 -- PECM2/LConn1

== system main_WU_motion/humerus ==
  body : sm_lib/Body Elements/File Solid  ExtGeomFileName=bones/humerus.obj  UnitType=Custom  ExtGeomFileUnits=m  StepReaderType=HEX  ExportConvexHullGeometry=off  InertiaType=Custom  Mass=m(3)  MassUnits=kg  CenterOfMass=hcom  CenterOfMassUnits=m  MomentsOfInertia=hI(1:3)  MomentsOfInertiaUnits=kg*m^2  ProductsOfInertia=hI(4:6)  ProductsOfInertiaUnits=kg*m^2  BasedOnType=Density  Density=1850  DensityUnits=kg/m^3  DoExposeReferenceFrame=on  SerializedFrames=<Frames/>  GraphicType=FromGeometry  MarkerShape=Sphere  MarkerSize=10  GraphicVisPropType=SimpleVisualProperties  GraphicDiffuseColor=[0.5 0.5 0.5]  GraphicSpecularColor=[0.5 0.5 0.5 1.0]  GraphicAmbientColor=[0.15 0.15 0.15 1.0]  GraphicEmissiveColor=[0.0 0.0 0.0 1.0]  GraphicShininess=75  GraphicOpacity=1.0
  H : PMIOPort  Side=Left
  connections:
  body/RConn1 -- H/RConn1

== system main_WU_motion/scapula ==
  body : sm_lib/Body Elements/File Solid  ExtGeomFileName=bones/scapula.obj  UnitType=Custom  ExtGeomFileUnits=m  StepReaderType=HEX  ExportConvexHullGeometry=off  InertiaType=Custom  Mass=m(2)  MassUnits=kg  CenterOfMass=scom  CenterOfMassUnits=m  MomentsOfInertia=sI(1:3)  MomentsOfInertiaUnits=kg*m^2  ProductsOfInertia=sI(4:6)  ProductsOfInertiaUnits=kg*m^2  BasedOnType=Density  Density=1850  DensityUnits=kg/m^3  DoExposeReferenceFrame=on  SerializedFrames=<Frames><Frame><Id>Frame1</Id><Value><Name>COM</Name><Origin><Source>CenterOfMassFrame</Source><FeatureName></FeatureName></Origin><PrimaryAxis><DefinedDirection>+Z</DefinedDirection><Source>ReferenceFrame</Source><SourceDirection>+Z</SourceDirection><FeatureName></FeatureName></PrimaryAxis><SecondaryAxis><DefinedDirection>+X</DefinedDirection><Source>ReferenceFrame</Source><SourceDirection>+X</SourceDirection><FeatureName></FeatureName></SecondaryAxis></Value></Frame></Frames>  GraphicType=FromGeometry  MarkerShape=Sphere  MarkerSize=10  GraphicVisPropType=SimpleVisualProperties  GraphicDiffuseColor=[0.5 0.5 0.5]  GraphicSpecularColor=[0.5 0.5 0.5 1.0]  GraphicAmbientColor=[0.15 0.15 0.15 1.0]  GraphicEmissiveColor=[0.0 0.0 0.0 1.0]  GraphicShininess=75  GraphicOpacity=1.0
  S : PMIOPort  Side=Right
  CoM : PMIOPort  Port=2  Side=Right
  connections:
  body/RConn1 -- S/RConn1
  CoM/RConn1 -- body/LConn1

== system main_WU_motion/scapulohumeral_rhythm ==
  1_point_contact : Subsystem  Commented=on
  2_points_contact : Subsystem  Commented=on
  Subsystem : Subsystem
  body_E : sm_lib/Body Elements/Spherical Solid  Commented=on  GraphicAmbientColor=[0.15 0.15 0.15 1.0]  BasedOnType=Mass  CenterOfMass=[0 0 0]  CenterOfMassUnits=m  GraphicDiffuseColor=[1 0 0]  Density=1000  DensityUnits=kg/m^3  DoExposeReferenceFrame=on  GraphicEmissiveColor=[0.0 0.0 0.0 1.0]  ExportEntireGeometry=off  SerializedExposedGeometries=<ExposedGeometries/>  SerializedFrames=<Frames/>  MarkerShape=Sphere  MarkerSize=10  GraphicType=FromGeometry  InertiaType=CalculateFromGeometry  Mass=0.001  MassUnits=kg  MomentsOfInertia=[1 1 1]  MomentsOfInertiaUnits=kg*m^2  GraphicOpacity=1.0  ProductsOfInertia=[0 0 0]  ProductsOfInertiaUnits=kg*m^2  GraphicShininess=75  GraphicSpecularColor=[0.5 0.5 0.5 1.0]  SphereRadius=0.05*r_ej  SphereRadiusUnits=m  GraphicVisPropType=SimpleVisualProperties
  body_ej : sm_lib/Body Elements/Ellipsoidal Solid  GraphicAmbientColor=[0.15 0.15 0.15 1.0]  BasedOnType=Density  CenterOfMass=[0 0 0]  CenterOfMassUnits=m  GraphicDiffuseColor=[1 0 0]  Density=1000  DensityUnits=kg/m^3  DoExposeReferenceFrame=on  EllipsoidRadii="[r_ej h_ej  r_ej]"  EllipsoidRadiiUnits=m  GraphicEmissiveColor=[0.0 0.0 0.0 1.0]  ExportEntireGeometry=off  SerializedFrames=<Frames/>  MarkerShape=Sphere  MarkerSize=10  GraphicType=FromGeometry  InertiaType=PointMass  Mass=0.001  MassUnits=kg  MomentsOfInertia=[1 1 1]  MomentsOfInertiaUnits=kg*m^2  GraphicOpacity=0.2  ProductsOfInertia=[0 0 0]  ProductsOfInertiaUnits=kg*m^2  GraphicShininess=75  GraphicSpecularColor=[0.5 0.5 0.5 1.0]  GraphicVisPropType=SimpleVisualProperties
  rot_x mu_ej : sm_lib/Frames and Transforms/Rigid Transform  TranslationMethod=None  TranslationStandardOffset=0  TranslationStandardOffsetUnits=m  TranslationStandardAxis=+Z  TranslationCartesianOffset=[0 0 0]  TranslationCartesianOffsetUnits=m  TranslationROffset=0  TranslationROffsetUnits=m  TranslationZOffset=0  TranslationZOffsetUnits=m  TranslationThetaOffset=0  TranslationThetaOffsetUnits=deg  RotationMethod=StandardAxis  RotationAngleUnits=deg  RotationStandardAxis=+X  RotationAngle=mu_ej  RotationArbitraryAxis=[0 0 1]  FollAlignAxisA=+X  BaseAlignAxisA=+Y  FollAlignAxisB=+Y  BaseAlignAxisB=+Z  RotationSequenceAxes=FollowerAxes  RotationSequence=XYX  RotationSequenceAngles=[0 0 0]  RotationSequenceAnglesUnits=deg  RotationMatrix=[1 0 0; 0 1 0; 0 0 1]  Quaternion=[1 0 0 0]
  rot_y phi_ej : sm_lib/Frames and Transforms/Rigid Transform  TranslationMethod=None  TranslationStandardOffset=0  TranslationStandardOffsetUnits=m  TranslationStandardAxis=+Z  TranslationCartesianOffset=[0 0 0]  TranslationCartesianOffsetUnits=m  TranslationROffset=0  TranslationROffsetUnits=m  TranslationZOffset=0  TranslationZOffsetUnits=m  TranslationThetaOffset=0  TranslationThetaOffsetUnits=deg  RotationMethod=StandardAxis  RotationAngleUnits=deg  RotationStandardAxis=+Y  RotationAngle=phi_ej  RotationArbitraryAxis=[0 0 1]  FollAlignAxisA=+X  BaseAlignAxisA=+Y  FollAlignAxisB=+Y  BaseAlignAxisB=+Z  RotationSequenceAxes=FollowerAxes  RotationSequence=XYX  RotationSequenceAngles=[0 0 0]  RotationSequenceAnglesUnits=deg  RotationMatrix=[1 0 0; 0 1 0; 0 0 1]  Quaternion=[1 0 0 0]
  rot_y psi_ej : sm_lib/Frames and Transforms/Rigid Transform  TranslationMethod=None  TranslationStandardOffset=0  TranslationStandardOffsetUnits=m  TranslationStandardAxis=+Z  TranslationCartesianOffset=[0 0 0]  TranslationCartesianOffsetUnits=m  TranslationROffset=0  TranslationROffsetUnits=m  TranslationZOffset=0  TranslationZOffsetUnits=m  TranslationThetaOffset=0  TranslationThetaOffsetUnits=deg  RotationMethod=StandardAxis  RotationAngleUnits=deg  RotationStandardAxis=+Y  RotationAngle=psi_ej  RotationArbitraryAxis=[0 0 1]  FollAlignAxisA=+X  BaseAlignAxisA=+Y  FollAlignAxisB=+Y  BaseAlignAxisB=+Z  RotationSequenceAxes=FollowerAxes  RotationSequence=XYX  RotationSequenceAngles=[0 0 0]  RotationSequenceAnglesUnits=deg  RotationMatrix=[1 0 0; 0 1 0; 0 0 1]  Quaternion=[1 0 0 0]
  transl xyz_ej : sm_lib/Frames and Transforms/Rigid Transform  TranslationMethod=Cartesian  TranslationStandardOffset=0  TranslationStandardOffsetUnits=m  TranslationStandardAxis=+Z  TranslationCartesianOffset=[x_ej y_ej z_ej]  TranslationCartesianOffsetUnits=m  TranslationROffset=0  TranslationROffsetUnits=m  TranslationZOffset=0  TranslationZOffsetUnits=m  TranslationThetaOffset=0  TranslationThetaOffsetUnits=deg  RotationMethod=None  RotationAngleUnits=deg  RotationStandardAxis=+Z  RotationAngle=0.0  RotationArbitraryAxis=[0 0 1]  FollAlignAxisA=+X  BaseAlignAxisA=+Y  FollAlignAxisB=+Y  BaseAlignAxisB=+Z  RotationSequenceAxes=FollowerAxes  RotationSequence=XYX  RotationSequenceAngles=[0 0 0]  RotationSequenceAnglesUnits=deg  RotationMatrix=[1 0 0; 0 1 0; 0 0 1]  Quaternion=[1 0 0 0]
  wf : PMIOPort  Side=Left
  S : PMIOPort  Port=2  Side=Right
  contact force : Outport
  wires:
  Subsystem/1(contact force) -> contact force/1
  connections:
  transl xyz_ej/LConn1 -- Subsystem/LConn1 -- wf/RConn1
  rot_y psi_ej/LConn1 -- transl xyz_ej/RConn1
  rot_x mu_ej/LConn1 -- rot_y psi_ej/RConn1
  rot_y phi_ej/LConn1 -- rot_x mu_ej/RConn1
  rot_y phi_ej/RConn1 -- body_E/RConn1 -- 1_point_contact/LConn1 -- 2_points_contact/LConn1 -- body_ej/RConn1
  S/RConn1 -- Subsystem/RConn1 -- 1_point_contact/RConn1 -- 2_points_contact/RConn1

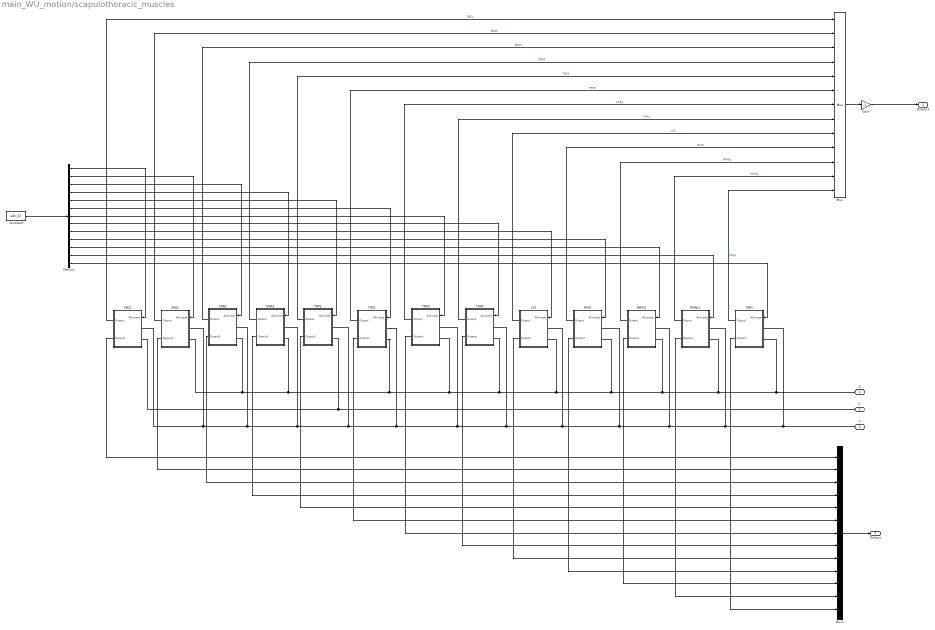
== system main_WU_motion/scapulothoracic_muscles ==
  Constant : Constant  Value=akt_ST
  Demux : Demux  Outputs=13
  Gain : Gain  Gain=-1
  LVS : Subsystem
  Mux : Mux  Inputs=13
  Mux1 : Mux  Inputs=13
  PMN : Subsystem
  RMN : Subsystem
  RMNJ1 : Subsystem
  RMNJ2 : Subsystem
  SBCL : Subsystem
  SRA1 : Subsystem
  SRA2 : Subsystem
  SRA3 : Subsystem
  TRP1 : Subsystem
  TRP2 : Subsystem
  TRP3 : Subsystem
  TRP4 : Subsystem
  S : PMIOPort  Side=Left
  C : PMIOPort  Port=2  Side=Left
  T : PMIOPort  Port=3  Side=Left
  Output : Outport
  Output1 : Outport  Port=2
  wires:
  TRP2/2(Output1) -> Mux1/6
  RMNJ2/2(Outport) -> Mux1/12
  SRA3/1(Output) -> Mux/4  "SRA3"
  TRP3/2(Outport) -> Mux1/7
  Mux1/1 -> Output/1
  SBCL/2(Output1) -> Mux1/1
  SRA1/2(Output1) -> Mux1/2
  TRP1/2(Output1) -> Mux1/5
  TRP2/1(Output) -> Mux/6  "TRP2"
  SRA2/2(Output1) -> Mux1/3
  SRA3/2(Output1) -> Mux1/4
  LVS/2(Outport) -> Mux1/9
  RMNJ1/2(Outport) -> Mux1/11
  LVS/1(Output) -> Mux/9  "LVS"
  PMN/1(Output) -> Mux/13  "PMIN"
  Mux/1 -> Gain/1
  RMNJ2/1(Output) -> Mux/12  "RMNJ2"
  TRP1/1(Output) -> Mux/5  "TRP1"
  TRP3/1(Output) -> Mux/7  "TRP3"
  RMNJ1/1(Output) -> Mux/11  "RMNJ1"
  SRA2/1(Output) -> Mux/3  "SRA2"
  SRA1/1(Output) -> Mux/2  "SRA1"
  TRP4/1(Output) -> Mux/8  "TRP4"
  RMN/1(Output) -> Mux/10  "RMN"
  TRP4/2(Outport) -> Mux1/8
  PMN/2(Outport) -> Mux1/13
  RMN/2(Outport) -> Mux1/10
  SBCL/1(Output) -> Mux/1  "SBCL"
  Gain/1 -> Output1/1
  Constant/1 -> Demux/1
  Demux/1 -> SBCL/1(Aktivace)
  Demux/2 -> SRA1/1(Aktivace)
  Demux/3 -> SRA2/1(Aktivace)
  Demux/4 -> SRA3/1(Aktivace)
  Demux/5 -> TRP1/1(Aktivace)
  Demux/6 -> TRP2/1(Aktivace)
  Demux/7 -> TRP3/1(Aktivace)
  Demux/8 -> TRP4/1(Aktivace)
  Demux/9 -> LVS/1(Aktivace)
  Demux/10 -> RMN/1(Aktivace)
  Demux/11 -> RMNJ1/1(Aktivace)
  Demux/12 -> RMNJ2/1(Aktivace)
  Demux/13 -> PMN/1(Aktivace)
  connections:
  SRA2/LConn1 -- SRA1/LConn1 -- SBCL/LConn1 -- SRA3/LConn1 -- TRP2/LConn1 -- TRP3/LConn1 -- TRP4/LConn1 -- LVS/LConn1 -- RMN/LConn1 -- RMNJ1/LConn1 -- RMNJ2/LConn1 -- PMN/LConn1 -- T/RConn1 -- TRP1/LConn1
  SRA3/LConn2 -- TRP3/LConn2 -- TRP4/LConn2 -- LVS/LConn2 -- RMN/LConn2 -- RMNJ1/LConn2 -- RMNJ2/LConn2 -- S/RConn1 -- PMN/LConn2 -- TRP2/LConn2 -- SRA2/LConn2 -- SRA1/LConn2
  SBCL/LConn2 -- C/RConn1 -- TRP1/LConn2

== system main_WU_motion/spine ==
  body : sm_lib/Body Elements/File Solid  ExtGeomFileName=bones\spine.obj  UnitType=Custom  ExtGeomFileUnits=m  StepReaderType=HEX  ExportConvexHullGeometry=off  InertiaType=CalculateFromGeometry  Mass=1  MassUnits=kg  CenterOfMass=[0 0 0]  CenterOfMassUnits=m  MomentsOfInertia=[1 1 1]  MomentsOfInertiaUnits=kg*m^2  ProductsOfInertia=[0 0 0]  ProductsOfInertiaUnits=kg*m^2  BasedOnType=Density  Density=1850  DensityUnits=kg/m^3  DoExposeReferenceFrame=on  SerializedFrames=<Frames/>  GraphicType=FromGeometry  MarkerShape=Sphere  MarkerSize=10  GraphicVisPropType=SimpleVisualProperties  GraphicDiffuseColor=[0.5 0.5 0.5]  GraphicSpecularColor=[0.5 0.5 0.5 1.0]  GraphicAmbientColor=[0.15 0.15 0.15 1.0]  GraphicEmissiveColor=[0.0 0.0 0.0 1.0]  GraphicShininess=75  GraphicOpacity=1.0
  R : PMIOPort  Side=Left
  connections:
  R/RConn1 -- body/RConn1

== system main_WU_motion/thorax ==
  body : sm_lib/Body Elements/File Solid  ExtGeomFileName=bones\thorax.obj  UnitType=Custom  ExtGeomFileUnits=m  StepReaderType=HEX  ExportConvexHullGeometry=off  InertiaType=CalculateFromGeometry  Mass=1  MassUnits=kg  CenterOfMass=[0 0 0]  CenterOfMassUnits=m  MomentsOfInertia=[1 1 1]  MomentsOfInertiaUnits=kg*m^2  ProductsOfInertia=[0 0 0]  ProductsOfInertiaUnits=kg*m^2  BasedOnType=Density  Density=1850  DensityUnits=kg/m^3  DoExposeReferenceFrame=on  SerializedFrames=<Frames/>  GraphicType=FromGeometry  MarkerShape=Sphere  MarkerSize=10  GraphicVisPropType=SimpleVisualProperties  GraphicDiffuseColor=[0.5 0.5 0.5]  GraphicSpecularColor=[0.5 0.5 0.5 1.0]  GraphicAmbientColor=[0.15 0.15 0.15 1.0]  GraphicEmissiveColor=[0.0 0.0 0.0 1.0]  GraphicShininess=75  GraphicOpacity=1.0
  R : PMIOPort  Side=Left
  connections:
  R/RConn1 -- body/RConn1
